simulink model "final_model"  (R2018a)
settings: Solver=VariableStepAuto  StartTime=0.0  StopTime=100  RelTol=1e-04
libraries: simulink x2
settings Model: Creator=geraldlow  LastModifiedBy=geraldlow
settings DebuggingCC: LibraryContextMissingDiagnostic=warning
settings SFSimCC: SimUseLocalCustomCode=on
settings RTWCC: RTWUseLocalCustomCode=on

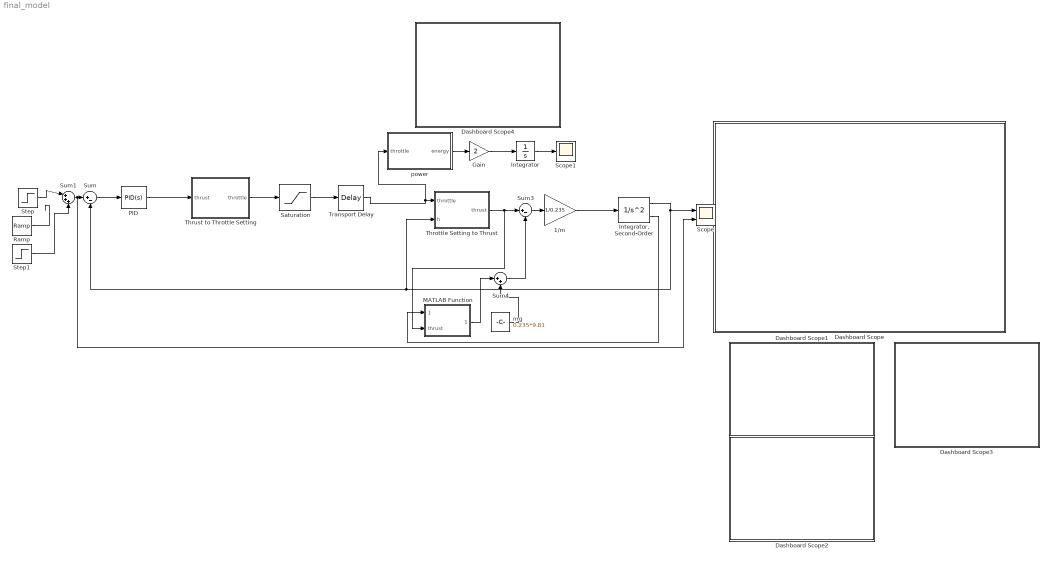
== system final_model ==
  1/m : Gain  Gain=1/0.235
  Dashboard Scope : Subsystem  DialogController=hmiCreateDDGDialog  IsWebBlock=on  mask(MWDashboardBlock){webBlockId=7af54a29-d889-46f3-93b8-2fd5d31388b0, webBlockType=sdiscope, ShowInLibBrowser=on, ShowInitialText=on, HMISrcModelName=final_model}
      mask prompts: webBlockId "WebBlock Id"; webBlockType "WebBlock Type"; HMISrcModelName "Source Model"
      mask help: Traces signals on the dashboard scope during simulation.
      mask Help: helpview([docroot '/mapfiles/simulink.map'], 'hmi_scope')
      mask Display:
      | if strcmp(get_param(bdroot(gcb),'BlockDiagramType'),'library')
      |  image([(matlabroot) '/toolbox/simulink/hmi/icons/SDIScope.png'])
      | end
  Dashboard Scope1 : Subsystem  DialogController=hmiCreateDDGDialog  IsWebBlock=on  mask(MWDashboardBlock){webBlockId=43b3c499-ead6-4af2-85a6-d1a124eeec5b, webBlockType=sdiscope, ShowInLibBrowser=on, ShowInitialText=on, HMISrcModelName=final_model}
      mask prompts: webBlockId "WebBlock Id"; webBlockType "WebBlock Type"; HMISrcModelName "Source Model"
      mask help: Traces signals on the dashboard scope during simulation.
      mask Help: helpview([docroot '/mapfiles/simulink.map'], 'hmi_scope')
      mask Display:
      | if strcmp(get_param(bdroot(gcb),'BlockDiagramType'),'library')
      |  image([(matlabroot) '/toolbox/simulink/hmi/icons/SDIScope.png'])
      | end
  Dashboard Scope2 : Subsystem  DialogController=hmiCreateDDGDialog  IsWebBlock=on  mask(MWDashboardBlock){webBlockId=b0764f20-5bcb-43e2-b85d-1a2044c39944, webBlockType=sdiscope, ShowInLibBrowser=on, ShowInitialText=on, HMISrcModelName=final_model}
      mask prompts: webBlockId "WebBlock Id"; webBlockType "WebBlock Type"; HMISrcModelName "Source Model"
      mask help: Traces signals on the dashboard scope during simulation.
      mask Help: helpview([docroot '/mapfiles/simulink.map'], 'hmi_scope')
      mask Display:
      | if strcmp(get_param(bdroot(gcb),'BlockDiagramType'),'library')
      |  image([(matlabroot) '/toolbox/simulink/hmi/icons/SDIScope.png'])
      | end
  Dashboard Scope3 : Subsystem  DialogController=hmiCreateDDGDialog  IsWebBlock=on  mask(MWDashboardBlock){webBlockId=21189764-3e5a-484c-aed0-6f95214b885e, webBlockType=sdiscope, ShowInLibBrowser=on, ShowInitialText=on, HMISrcModelName=final_model}
      mask prompts: webBlockId "WebBlock Id"; webBlockType "WebBlock Type"; HMISrcModelName "Source Model"
      mask help: Traces signals on the dashboard scope during simulation.
      mask Help: helpview([docroot '/mapfiles/simulink.map'], 'hmi_scope')
      mask Display:
      | if strcmp(get_param(bdroot(gcb),'BlockDiagramType'),'library')
      |  image([(matlabroot) '/toolbox/simulink/hmi/icons/SDIScope.png'])
      | end
  Dashboard Scope4 : Subsystem  DialogController=hmiCreateDDGDialog  IsWebBlock=on  mask(MWDashboardBlock){webBlockId=23f3d4c3-c494-4d8d-9901-5459374ed13a, webBlockType=sdiscope, ShowInLibBrowser=on, ShowInitialText=on, HMISrcModelName=final_model}
      mask prompts: webBlockId "WebBlock Id"; webBlockType "WebBlock Type"; HMISrcModelName "Source Model"
      mask help: Traces signals on the dashboard scope during simulation.
      mask Help: helpview([docroot '/mapfiles/simulink.map'], 'hmi_scope')
      mask Display:
      | if strcmp(get_param(bdroot(gcb),'BlockDiagramType'),'library')
      |  image([(matlabroot) '/toolbox/simulink/hmi/icons/SDIScope.png'])
      | end
  Gain : Gain  Gain=2
  Integrator : Integrator
  "Integrator, Second-Order" : SecondOrderIntegrator  ICX=0  LimitX=on  LowerLimitX=0
  MATLAB Function : MATLAB Function  TreatAsAtomicUnit=on
  PID : simulink/Continuous/PID Controller  Controller=PID  Form=Parallel  TimeDomain=Continuous-time  SampleTime=-1  IntegratorMethod=Forward Euler  FilterMethod=Forward Euler  ControllerParametersSource=internal  P=.2  I=1.3e-01  D=1.8  UseFilter=on  N=78.67  TunerSelectOption=Transfer Function Based (PID Tuner App)  InitialConditionSource=internal  InitialConditionForIntegrator=0  InitialConditionForFilter=0  DifferentiatorICPrevScaledInput=0  ExternalReset=none  TrackingMode=off  Kt=1  LimitOutput=off  UpperSaturationLimit=inf  LowerSaturationLimit=-inf  LinearizeAsGain=on  AntiWindupMode=none  Kb=1  POutMin=[]  POutMax=[]  IOutMin=[]  IOutMax=[]  DOutMin=[]  DOutMax=[]  NOutMin=[]  NOutMax=[]  SumOutMin=[]  SumOutMax=[]  SaturationOutMin=[]  SaturationOutMax=[]  PParamMin=[]  PParamMax=[]  IParamMin=[]  IParamMax=[]  DParamMin=[]  DParamMax=[]  NParamMin=[]  NParamMax=[]  KbParamMin=[]  KbParamMax=[]  KtParamMin=[]  KtParamMax=[]  KbOutMin=[]  KbOutMax=[]  KtOutMin=[]  KtOutMax=[]  IntegratorOutMin=[]  IntegratorOutMax=[]  FilterOutMin=[]  FilterOutMax=[]  SumI1OutMin=[]  SumI1OutMax=[]  SumI2OutMin=[]  SumI2OutMax=[]  SumI3OutMin=[]  SumI3OutMax=[]  SumDOutMin=[]  SumDOutMax=[]  DifferentiatorOutMin=[]  DifferentiatorOutMax=[]  FilterDiffOutCoefMin=[]  FilterDiffOutCoefMax=[]  ReciprocalOutMin=[]  ReciprocalOutMax=[]  SumDenOutMin=[]  SumDenOutMax=[]  SumNumOutMin=[]  SumNumOutMax=[]  DivideOutMin=[]  DivideOutMax=[]  IntegratorContinuousStateAttributes=''  IntegratorStateMustResolveToSignalObject=off  IntegratorRTWStateStorageClass=Auto  FilterContinuousStateAttributes=''  FilterStateMustResolveToSignalObject=off  FilterRTWStateStorageClass=Auto
  Ramp : simulink/Sources/Ramp  slope=.125  start=15  InitialOutput=0
  Saturation : Saturate  UpperLimit=100  LowerLimit=0
  Scope : Scope  NumInputPorts=2
  Scope1 : Scope
  Step : Step  Time=10  After=.7  SampleTime=0
  Step1 : Step  Time=20  After=.5  SampleTime=0
  Sum : Sum  Inputs=|+-
  Sum1 : Sum  Inputs=|+++
  Sum3 : Sum  Inputs=|+-
  Sum4 : Sum  Inputs=|++
  Throttle Setting to Thrust : MATLAB Function  TreatAsAtomicUnit=on
  Thrust to Throttle Setting : MATLAB Function  TreatAsAtomicUnit=on
  Transport Delay : TransportDelay  DelayTime=.2
  mg : Constant  Value=0.235*9.81
  power : MATLAB Function  TreatAsAtomicUnit=on
  wires:
  Sum/1 -> PID/1
  Thrust to Throttle Setting/1(throttle) -> Saturation/1
  mg/1 -> Sum4/2
  Sum3/1 -> 1/m/1
  "Integrator, Second-Order"/1 -> Scope/1, Sum/2, Throttle Setting to Thrust/2(h)
  Sum1/1 -> Sum/1, Scope/2
  Sum4/1 -> Sum3/2
  MATLAB Function/1(friction) -> Sum4/1
  Throttle Setting to Thrust/1(thrust) -> MATLAB Function/2(thrust), Sum3/1
  1/m/1 -> "Integrator, Second-Order"/1
  Ramp/1 -> ?
  PID/1 -> Thrust to Throttle Setting/1(thrust)
  Step/1 -> Sum1/1
  Step1/1 -> Sum1/3
  Integrator/1 -> Scope1/1
  power/1(energy) -> Gain/1
  Gain/1 -> Integrator/1
  "Integrator, Second-Order"/2 -> MATLAB Function/1(velocity)
  Saturation/1 -> Transport Delay/1
  Transport Delay/1 -> Throttle Setting to Thrust/1(throttle), power/1(throttle)

== system final_model/Dashboard Scope ==

== system final_model/Dashboard Scope1 ==

== system final_model/Dashboard Scope2 ==

== system final_model/Dashboard Scope3 ==

== system final_model/Dashboard Scope4 ==

== matlab function final_model/Throttle Setting to Thrust ==
  data: throttle input; thrust output; h input
function thrust = fcn(throttle, h)
r=0.1524;
if throttle < 1
   thrust = 0;
elseif throttle > 88
   thrust=2*9.81*.66;
else
   thrust=2*9.81*(0.1+(.66-0.1)/(88-1)*(throttle-1));
end

   h=h+0.05;
   thrust=thrust/(1-r^2/(16*h^2))-h*r^2/(2*sqrt(4*h^2)^3);
end

== matlab function final_model/Thrust to Throttle Setting ==
  data: thrust input; throttle output
function throttle = fcn(thrust)
% (.66-0.1)/(88-1)*2*9.81 = 0.1263
throttle = (thrust / 0.1263)+.8;
end

== matlab function final_model/MATLAB Function ==
  data: velocity input; friction output; thrust input
function friction   = fcn(velocity, thrust)
epsilon = 0.005; %small perturbation
mg = 0.235*9.81;
% Get reasonable values for x1, x2, l
x1 = 0.0125;
x2 = 0.0125;
l = 0.221;
netforce = thrust-mg; %mg should be a constant defined.
mu = 0.15; %coeff of dynamic friction
%static friction
if abs(velocity) < epsilon && abs(netforce) < 0.13*9.81 && netforce > 0
    friction = netforce;
elseif abs(velocity) < epsilon && abs(netforce) < 0.13*9.81 && netforce < 0
    friction = -netforce;
elseif velocity > 0
    friction=2*mu*(mg*x1-thrust*x2)/l;
elseif velocity < 0
    friction=-2*mu*(mg*x1-thrust*x2)/l;
else
    friction=0;
end

== matlab function final_model/power ==
  data: throttle input; energy output
function energy =power(throttle)
epsilon=0.001;
if throttle<epsilon
    energy=0;
elseif throttle<90

energy=(500-10)/90*throttle+10;
else
    energy=200;
end
end
